simulink model "LQR"  (R2015a)
settings: Solver=ode45  StartTime=0.0  StopTime=20  RelTol=1e-3
undefined symbols (not defined in the file): A, B, C, kf, Kp, L
settings Model: CovSFcnEnable=off  Creator=jordan  LastModifiedBy=Vladislav
settings DebuggingCC: SolverPrmCheckMsg=warning

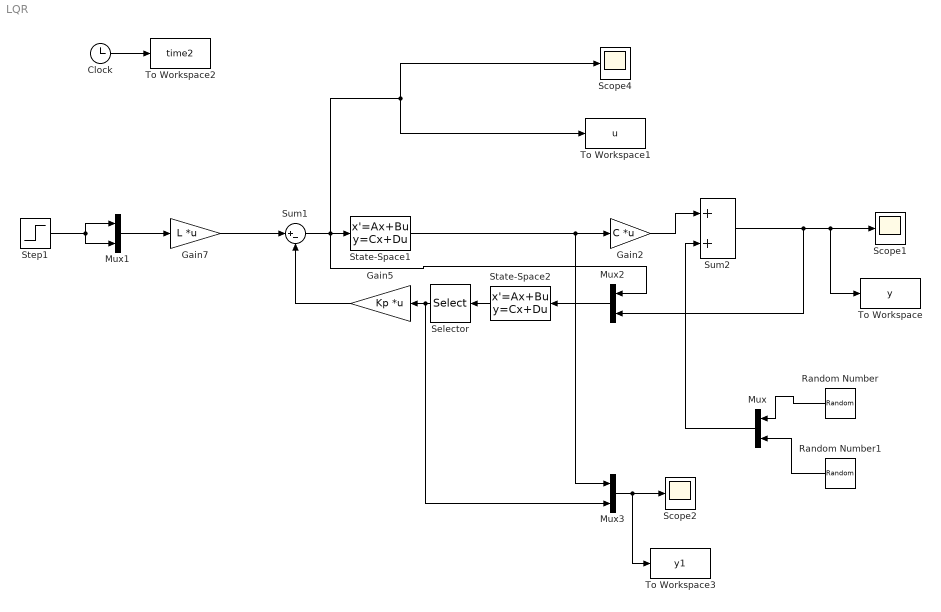
== system LQR ==
  Clock : Clock
  Gain2 : Gain  Gain=C  Multiplication=Matrix(K*u)
  Gain5 : Gain  Gain=Kp  Multiplication=Matrix(K*u)
  Gain7 : Gain  Gain=L  Multiplication=Matrix(K*u)
  Mux{,1..3} (4 alike) : Mux  Inputs=2
  Random Number : RandomNumber  Variance=0.01  SampleTime=0.1
  Random Number1 : RandomNumber  Variance=0.01  Seed=1  SampleTime=0.1
  Scope1 : Scope
      settings: TimeRange=10  YMin=-0.2  YMax=1.2
  Scope2 : Scope
      settings: TimeRange=10  YMin=-0.2  YMax=1.2  SaveName=ScopeData2
  Scope4 : Scope
      settings: TimeRange=10  YMin=-0.2  YMax=1.4
  Selector : Selector  InputPortWidth=6  Indices=[3:6]
  State-Space1 : StateSpace  A=A  B=B  C=eye(4)  D=zeros(4,2)  X0=0
  State-Space2 : StateSpace  A=kf.a  B=kf.b  C=kf.c  D=kf.d  X0=0
  Step1 : Step  Time=0  SampleTime=0
  Sum1 : Sum  Inputs=|+-
  Sum2 : Sum  Inputs=|++
  To Workspace : ToWorkspace  VariableName=y  SampleTime=-1
  To Workspace1 : ToWorkspace  VariableName=u  SampleTime=-1
  To Workspace2 : ToWorkspace  VariableName=time2  SampleTime=-1
  To Workspace3 : ToWorkspace  VariableName=y1  SampleTime=-1
  wires:
  Gain7/1 -> Sum1/1
  Step1/1 -> Mux1/1, Mux1/2
  Mux1/1 -> Gain7/1
  State-Space1/1 -> Mux3/1, Gain2/1
  Clock/1 -> To Workspace2/1
  Random Number1/1 -> Mux/2
  Random Number/1 -> Mux/1
  State-Space2/1 -> Selector/1
  Mux2/1 -> State-Space2/1
  Sum1/1 -> Mux2/1, State-Space1/1, To Workspace1/1, Scope4/1
  Gain5/1 -> Sum1/2
  Selector/1 -> Mux3/2, Gain5/1
  Gain2/1 -> Sum2/1
  Sum2/1 -> Mux2/2, To Workspace/1, Scope1/1
  Mux/1 -> Sum2/2
  Mux3/1 -> To Workspace3/1, Scope2/1
